simulink model "FirstModel"  (R2020a)
settings: Solver=VariableStepAuto  StartTime=0.0  StopTime=10.0  RelTol=1e-3
settings Model: Creator=Mohammad  LastModifiedBy=Mohammad

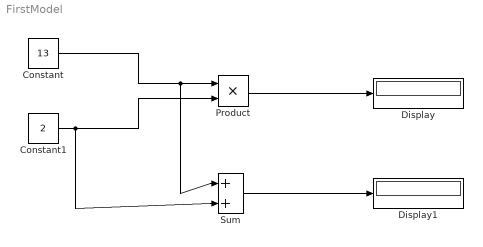
== system FirstModel ==
  Constant : Constant  Value=13
  Constant1 : Constant  Value=2
  Display : Display
  Display1 : Display
  Product : Product
  Sum : Sum  Inputs=|++
  wires:
  Constant1/1 -> Sum/2, Product/2
  Constant/1 -> Sum/1, Product/1
  Product/1 -> Display/1
  Sum/1 -> Display1/1
